simulink model "punto_e1"  (R2014a)
settings: Solver=ode45  StartTime=0.0  StopTime=50.0  RelTol=1e-3
values from neighbouring files (symbols this model uses):
  Kc = 1    [es1.m]
  Kr = 1    [es1.m]
libraries: cstblocks x1, simulink x1
settings Model: Creator=HP  LastModifiedBy=HP

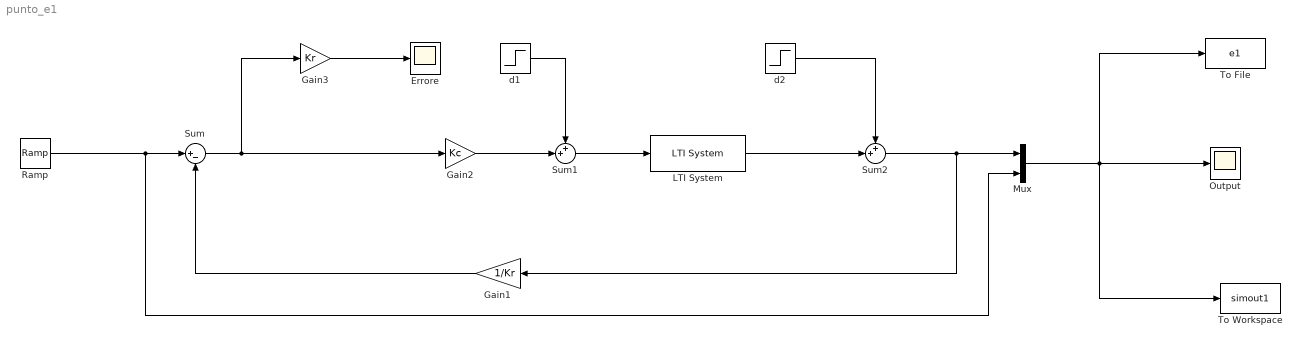
== system punto_e1 ==
  Errore : Scope
  Gain1 : Gain  Gain=1/Kr
  Gain2 : Gain  Gain=Kc
  Gain3 : Gain  Gain=Kr
  LTI System : cstblocks/LTI System  sys=F  IC=[]
  Mux : Mux  Inputs=2
  Output : Scope
  Ramp : simulink/Sources/Ramp  slope=1  start=0  X0=0
  Sum : Sum  Inputs=|+-
  Sum1 : Sum  Inputs=++|
  Sum2 : Sum  Inputs=++|
  To File : ToFile  Filename=e1  MatrixName=output  SaveFormat=Timeseries
  To Workspace : ToWorkspace  VariableName=simout1  SaveFormat=Timeseries  SampleTime=-1
  d1 : Step  Time=0  After=0.1  SampleTime=0
  d2 : Step  Time=0  After=0.5  SampleTime=0
  wires:
  Sum/1 -> Gain3/1, Gain2/1
  Gain1/1 -> Sum/2
  d1/1 -> Sum1/1
  Gain2/1 -> Sum1/2
  Sum1/1 -> LTI System/1
  LTI System/1 -> Sum2/2
  d2/1 -> Sum2/1
  Sum2/1 -> Gain1/1, Mux/1
  Mux/1 -> To File/1, To Workspace/1, Output/1
  Ramp/1 -> Mux/2, Sum/1
  Gain3/1 -> Errore/1
